simulink model "VehCtrl20260630_18B"  (R2018b)
settings: Solver=FixedStepAuto  StartTime=0.0  StopTime=inf  FixedStep=0.005  RelTol=1e-3
InitFcn:
  | mbd_mpc_consistency_checks(bdroot(gcs));
undefined symbols (not defined in the file): ANG_DEAD, BMS_NormalPwr, BrakeDeadZone, BrkPrsByBrkPct_TB_X, BrkPrsByBrkPct_TB_Y, DELAY_DISCHARGE, DELAY_RCUOFF, DRV_BACKWARD, DRV_BRAKE, DRV_FORWARD, DRV_NEUTRAL, DRV_PARK, DRV_UNPARK, DRV_ZEROTURN, EPB_LOCK, EPB_UNLOCK, ExtraLoadPwr, FanOff, fifo_0_vect, fifo_1_vect, HiFanReq, HV_finished, HV_No_Active, HV_POWER_OFF, HV_POWER_ON, HVDown, HVON, KaTLS_v_DrgUp_X_VehSpd, KeFTM_s_Way1OffDlyTime, KeFTM_TK_Way1CoolLv2OffBatTemp, KeFTM_TK_Way1CoolLv2OffMtrTemp, KeFTM_TK_Way1CoolLv2OnBatTemp, KeFTM_TK_Way1CoolLv2OnMtrTemp, KeFTM_TK_Way1CoolLv3OffBatTemp, KeFTM_TK_Way1CoolLv3OffMtrTemp, KeFTM_TK_Way1CoolLv3OnBatTemp, KeFTM_TK_Way1CoolLv3OnMtrTemp, KeFTM_TK_Way1CoolLv4OffBatTemp, KeFTM_TK_Way1CoolLv4OffMtrTemp, KeFTM_TK_Way1CoolLv4OnBatTemp, KeFTM_TK_Way1CoolLv4OnMtrTemp, Kp1, Kp2, LowFanReq, LQFP, MtrCmdGainFL, MtrCmdGainFR, MtrCmdGainRL, MtrCmdGainRR, MtrPwrFactor_RCU, MtrPwrHighToMidThd, MtrPwrLowToMidThd, MtrPwrMidToHighThd, MtrPwrMidToLowThd, MtrTrqMax, PCT_DEAD, Precharge, PTO_1000, PTO_540, pts1_fifo_0_vect ... (+32)
libraries: mbd_mpc574x_ec_toolbox x175, simulink x110, canmsglib x70
(part 6 of 15)

== system VehCtrl20260630_18B/SigIn/CAN0/RMT_VCU4 ==
  ID : Inport
  Data : Inport  Port=2
  length : Inport  Port=3
  timestamp : Inport  Port=4
  Switch Case : SwitchCase  CaseConditions={hex2dec('4')}  ShowDefaultCase=off
  UNPACK : Subsystem  TreatAsAtomicUnit=on
  Message : Outport
  wires:
  Switch Case/1 -> UNPACK/Action
  ID/1 -> UNPACK/1(ID), Switch Case/1
  Data/1 -> UNPACK/2(data)
  timestamp/1 -> UNPACK/4(timestamp)
  length/1 -> UNPACK/3(length)
  UNPACK/1(Message) -> Message/1

== system VehCtrl20260630_18B/SigIn/CAN1/ACM_Msg ==
  ID : Inport
  Data : Inport  Port=2
  length : Inport  Port=3
  timestamp : Inport  Port=4
  Switch Case : SwitchCase  CaseConditions={hex2dec('284')}  ShowDefaultCase=off
  UNPACK : Subsystem  TreatAsAtomicUnit=on
  Message : Outport
  wires:
  Switch Case/1 -> UNPACK/Action
  ID/1 -> UNPACK/1(ID), Switch Case/1
  Data/1 -> UNPACK/2(data)
  timestamp/1 -> UNPACK/4(timestamp)
  length/1 -> UNPACK/3(length)
  UNPACK/1(Message) -> Message/1

== system VehCtrl20260630_18B/SigIn/CAN1/AVCU_Msg ==
  ID : Inport
  Data : Inport  Port=2
  length : Inport  Port=3
  timestamp : Inport  Port=4
  Switch Case : SwitchCase  CaseConditions={hex2dec('180')}  ShowDefaultCase=off
  UNPACK : Subsystem  TreatAsAtomicUnit=on
  Message : Outport
  wires:
  UNPACK/1(Message) -> Message/1
  length/1 -> UNPACK/3(length)
  timestamp/1 -> UNPACK/4(timestamp)
  Data/1 -> UNPACK/2(data)
  ID/1 -> Switch Case/1, UNPACK/1(ID)
  Switch Case/1 -> UNPACK/Action

== system VehCtrl20260630_18B/SigIn/CAN1/BMS_CANWakeUpID ==
  ID : Inport
  Data : Inport  Port=2
  length : Inport  Port=3
  timestamp : Inport  Port=4
  Switch Case : SwitchCase  CaseConditions={hex2dec('180D2947')}  ShowDefaultCase=off
  UNPACK : Subsystem  TreatAsAtomicUnit=on
  Message : Outport
  wires:
  UNPACK/1(Message) -> Message/1
  length/1 -> UNPACK/3(length)
  timestamp/1 -> UNPACK/4(timestamp)
  Data/1 -> UNPACK/2(data)
  ID/1 -> Switch Case/1, UNPACK/1(ID)
  Switch Case/1 -> UNPACK/Action

== system VehCtrl20260630_18B/SigIn/CAN1/BMS_CellTempCycTx ==
  ID : Inport
  Data : Inport  Port=2
  length : Inport  Port=3
  timestamp : Inport  Port=4
  Switch Case : SwitchCase  CaseConditions={hex2dec('18602947')}  ShowDefaultCase=off
  UNPACK : Subsystem  TreatAsAtomicUnit=on
  Message : Outport
  wires:
  UNPACK/1(Message) -> Message/1
  length/1 -> UNPACK/3(length)
  timestamp/1 -> UNPACK/4(timestamp)
  Data/1 -> UNPACK/2(data)
  ID/1 -> Switch Case/1, UNPACK/1(ID)
  Switch Case/1 -> UNPACK/Action

== system VehCtrl20260630_18B/SigIn/CAN1/BMS_CellVoltageCycTx ==
  ID : Inport
  Data : Inport  Port=2
  length : Inport  Port=3
  timestamp : Inport  Port=4
  Switch Case : SwitchCase  CaseConditions={hex2dec('18202947')}  ShowDefaultCase=off
  UNPACK : Subsystem  TreatAsAtomicUnit=on
  Message : Outport
  wires:
  UNPACK/1(Message) -> Message/1
  length/1 -> UNPACK/3(length)
  timestamp/1 -> UNPACK/4(timestamp)
  Data/1 -> UNPACK/2(data)
  ID/1 -> Switch Case/1, UNPACK/1(ID)
  Switch Case/1 -> UNPACK/Action

== system VehCtrl20260630_18B/SigIn/CAN1/BMS_ExtremeCellVoltage ==
  ID : Inport
  Data : Inport  Port=2
  length : Inport  Port=3
  timestamp : Inport  Port=4
  Switch Case : SwitchCase  CaseConditions={hex2dec('18022947')}  ShowDefaultCase=off
  UNPACK : Subsystem  TreatAsAtomicUnit=on
  Message : Outport
  wires:
  UNPACK/1(Message) -> Message/1
  length/1 -> UNPACK/3(length)
  timestamp/1 -> UNPACK/4(timestamp)
  Data/1 -> UNPACK/2(data)
  ID/1 -> Switch Case/1, UNPACK/1(ID)
  Switch Case/1 -> UNPACK/Action

== system VehCtrl20260630_18B/SigIn/CAN1/BMS_ExtremeTemp ==
  ID : Inport
  Data : Inport  Port=2
  length : Inport  Port=3
  timestamp : Inport  Port=4
  Switch Case : SwitchCase  CaseConditions={hex2dec('18032947')}  ShowDefaultCase=off
  UNPACK : Subsystem  TreatAsAtomicUnit=on
  Message : Outport
  wires:
  UNPACK/1(Message) -> Message/1
  length/1 -> UNPACK/3(length)
  timestamp/1 -> UNPACK/4(timestamp)
  Data/1 -> UNPACK/2(data)
  ID/1 -> Switch Case/1, UNPACK/1(ID)
  Switch Case/1 -> UNPACK/Action

== system VehCtrl20260630_18B/SigIn/CAN1/BMS_PackCalc ==
  ID : Inport
  Data : Inport  Port=2
  length : Inport  Port=3
  timestamp : Inport  Port=4
  Switch Case : SwitchCase  CaseConditions={hex2dec('18052947')}  ShowDefaultCase=off
  UNPACK : Subsystem  TreatAsAtomicUnit=on
  Message : Outport
  wires:
  UNPACK/1(Message) -> Message/1
  length/1 -> UNPACK/3(length)
  timestamp/1 -> UNPACK/4(timestamp)
  Data/1 -> UNPACK/2(data)
  ID/1 -> Switch Case/1, UNPACK/1(ID)
  Switch Case/1 -> UNPACK/Action

== system VehCtrl20260630_18B/SigIn/CAN1/BMS_PackLimitPower ==
  ID : Inport
  Data : Inport  Port=2
  length : Inport  Port=3
  timestamp : Inport  Port=4
  Switch Case : SwitchCase  CaseConditions={hex2dec('18062947')}  ShowDefaultCase=off
  UNPACK : Subsystem  TreatAsAtomicUnit=on
  Message : Outport
  wires:
  Switch Case/1 -> UNPACK/Action
  ID/1 -> UNPACK/1(ID), Switch Case/1
  Data/1 -> UNPACK/2(data)
  timestamp/1 -> UNPACK/4(timestamp)
  length/1 -> UNPACK/3(length)
  UNPACK/1(Message) -> Message/1

== system VehCtrl20260630_18B/SigIn/CAN1/BMS_PackMeasure ==
  ID : Inport
  Data : Inport  Port=2
  length : Inport  Port=3
  timestamp : Inport  Port=4
  Switch Case : SwitchCase  CaseConditions={hex2dec('18012947')}  ShowDefaultCase=off
  UNPACK : Subsystem  TreatAsAtomicUnit=on
  Message : Outport
  wires:
  UNPACK/1(Message) -> Message/1
  length/1 -> UNPACK/3(length)
  timestamp/1 -> UNPACK/4(timestamp)
  Data/1 -> UNPACK/2(data)
  ID/1 -> Switch Case/1, UNPACK/1(ID)
  Switch Case/1 -> UNPACK/Action

== system VehCtrl20260630_18B/SigIn/CAN1/BMS_PackStateInf ==
  ID : Inport
  Data : Inport  Port=2
  length : Inport  Port=3
  timestamp : Inport  Port=4
  Switch Case : SwitchCase  CaseConditions={hex2dec('18042947')}  ShowDefaultCase=off
  UNPACK : Subsystem  TreatAsAtomicUnit=on
  Message : Outport
  wires:
  Switch Case/1 -> UNPACK/Action
  ID/1 -> UNPACK/1(ID), Switch Case/1
  Data/1 -> UNPACK/2(data)
  timestamp/1 -> UNPACK/4(timestamp)
  length/1 -> UNPACK/3(length)
  UNPACK/1(Message) -> Message/1

== system VehCtrl20260630_18B/SigIn/CAN1/BMS_Relaystatus ==
  ID : Inport
  Data : Inport  Port=2
  length : Inport  Port=3
  timestamp : Inport  Port=4
  Switch Case : SwitchCase  CaseConditions={hex2dec('1C1F7547')}  ShowDefaultCase=off
  UNPACK : Subsystem  TreatAsAtomicUnit=on
  Message : Outport
  wires:
  UNPACK/1(Message) -> Message/1
  length/1 -> UNPACK/3(length)
  timestamp/1 -> UNPACK/4(timestamp)
  Data/1 -> UNPACK/2(data)
  ID/1 -> Switch Case/1, UNPACK/1(ID)
  Switch Case/1 -> UNPACK/Action

== system VehCtrl20260630_18B/SigIn/CAN1/DbugBMS_ESM ==
  ID : Inport
  Data : Inport  Port=2
  length : Inport  Port=3
  timestamp : Inport  Port=4
  Switch Case : SwitchCase  CaseConditions={hex2dec('1C067547')}  ShowDefaultCase=off
  UNPACK : Subsystem  TreatAsAtomicUnit=on
  Message : Outport
  wires:
  UNPACK/1(Message) -> Message/1
  length/1 -> UNPACK/3(length)
  timestamp/1 -> UNPACK/4(timestamp)
  Data/1 -> UNPACK/2(data)
  ID/1 -> Switch Case/1, UNPACK/1(ID)
  Switch Case/1 -> UNPACK/Action

== system VehCtrl20260630_18B/SigIn/CAN1/DbugBMS_SOC_CaleSOC ==
  ID : Inport
  Data : Inport  Port=2
  length : Inport  Port=3
  timestamp : Inport  Port=4
  Switch Case : SwitchCase  CaseConditions={hex2dec('1C017547')}  ShowDefaultCase=off
  UNPACK : Subsystem  TreatAsAtomicUnit=on
  Message : Outport
  wires:
  Switch Case/1 -> UNPACK/Action
  ID/1 -> UNPACK/1(ID), Switch Case/1
  Data/1 -> UNPACK/2(data)
  timestamp/1 -> UNPACK/4(timestamp)
  length/1 -> UNPACK/3(length)
  UNPACK/1(Message) -> Message/1

== system VehCtrl20260630_18B/SigIn/CAN1/MCU2VCU_1 ==
  ID : Inport
  Data : Inport  Port=2
  length : Inport  Port=3
  timestamp : Inport  Port=4
  Switch Case : SwitchCase  CaseConditions={hex2dec('C08A7F3')}  ShowDefaultCase=off
  UNPACK : Subsystem  TreatAsAtomicUnit=on
  Message : Outport
  wires:
  Switch Case/1 -> UNPACK/Action
  ID/1 -> UNPACK/1(ID), Switch Case/1
  Data/1 -> UNPACK/2(data)
  timestamp/1 -> UNPACK/4(timestamp)
  length/1 -> UNPACK/3(length)
  UNPACK/1(Message) -> Message/1

== system VehCtrl20260630_18B/SigIn/CAN1/MCU2VCU_10 ==
  ID : Inport
  Data : Inport  Port=2
  length : Inport  Port=3
  timestamp : Inport  Port=4
  Switch Case : SwitchCase  CaseConditions={hex2dec('C09A7F0')}  ShowDefaultCase=off
  UNPACK : Subsystem  TreatAsAtomicUnit=on
  Message : Outport
  wires:
  Switch Case/1 -> UNPACK/Action
  ID/1 -> UNPACK/1(ID), Switch Case/1
  Data/1 -> UNPACK/2(data)
  timestamp/1 -> UNPACK/4(timestamp)
  length/1 -> UNPACK/3(length)
  UNPACK/1(Message) -> Message/1

== system VehCtrl20260630_18B/SigIn/CAN1/MCU2VCU_11 ==
  ID : Inport
  Data : Inport  Port=2
  length : Inport  Port=3
  timestamp : Inport  Port=4
  Switch Case : SwitchCase  CaseConditions={hex2dec('C0AA7F0')}  ShowDefaultCase=off
  UNPACK : Subsystem  TreatAsAtomicUnit=on
  Message : Outport
  wires:
  UNPACK/1(Message) -> Message/1
  length/1 -> UNPACK/3(length)
  timestamp/1 -> UNPACK/4(timestamp)
  Data/1 -> UNPACK/2(data)
  ID/1 -> Switch Case/1, UNPACK/1(ID)
  Switch Case/1 -> UNPACK/Action

== system VehCtrl20260630_18B/SigIn/CAN1/MCU2VCU_12 ==
  ID : Inport
  Data : Inport  Port=2
  length : Inport  Port=3
  timestamp : Inport  Port=4
  Switch Case : SwitchCase  CaseConditions={hex2dec('C0BA7F0')}  ShowDefaultCase=off
  UNPACK : Subsystem  TreatAsAtomicUnit=on
  Message : Outport
  wires:
  Switch Case/1 -> UNPACK/Action
  ID/1 -> UNPACK/1(ID), Switch Case/1
  Data/1 -> UNPACK/2(data)
  timestamp/1 -> UNPACK/4(timestamp)
  length/1 -> UNPACK/3(length)
  UNPACK/1(Message) -> Message/1

== system VehCtrl20260630_18B/SigIn/CAN1/MCU2VCU_13 ==
  ID : Inport
  Data : Inport  Port=2
  length : Inport  Port=3
  timestamp : Inport  Port=4
  Switch Case : SwitchCase  CaseConditions={hex2dec('C08A7F1')}  ShowDefaultCase=off
  UNPACK : Subsystem  TreatAsAtomicUnit=on
  Message : Outport
  wires:
  Switch Case/1 -> UNPACK/Action
  ID/1 -> UNPACK/1(ID), Switch Case/1
  Data/1 -> UNPACK/2(data)
  timestamp/1 -> UNPACK/4(timestamp)
  length/1 -> UNPACK/3(length)
  UNPACK/1(Message) -> Message/1

== system VehCtrl20260630_18B/SigIn/CAN1/MCU2VCU_14 ==
  ID : Inport
  Data : Inport  Port=2
  length : Inport  Port=3
  timestamp : Inport  Port=4
  Switch Case : SwitchCase  CaseConditions={hex2dec('C09A7F1')}  ShowDefaultCase=off
  UNPACK : Subsystem  TreatAsAtomicUnit=on
  Message : Outport
  wires:
  UNPACK/1(Message) -> Message/1
  length/1 -> UNPACK/3(length)
  timestamp/1 -> UNPACK/4(timestamp)
  Data/1 -> UNPACK/2(data)
  ID/1 -> Switch Case/1, UNPACK/1(ID)
  Switch Case/1 -> UNPACK/Action

== system VehCtrl20260630_18B/SigIn/CAN1/MCU2VCU_15 ==
  ID : Inport
  Data : Inport  Port=2
  length : Inport  Port=3
  timestamp : Inport  Port=4
  Switch Case : SwitchCase  CaseConditions={hex2dec('C0AA7F1')}  ShowDefaultCase=off
  UNPACK : Subsystem  TreatAsAtomicUnit=on
  Message : Outport
  wires:
  Switch Case/1 -> UNPACK/Action
  ID/1 -> UNPACK/1(ID), Switch Case/1
  Data/1 -> UNPACK/2(data)
  timestamp/1 -> UNPACK/4(timestamp)
  length/1 -> UNPACK/3(length)
  UNPACK/1(Message) -> Message/1

== system VehCtrl20260630_18B/SigIn/CAN1/MCU2VCU_16 ==
  ID : Inport
  Data : Inport  Port=2
  length : Inport  Port=3
  timestamp : Inport  Port=4
  Switch Case : SwitchCase  CaseConditions={hex2dec('C0BA7F1')}  ShowDefaultCase=off
  UNPACK : Subsystem  TreatAsAtomicUnit=on
  Message : Outport
  wires:
  UNPACK/1(Message) -> Message/1
  length/1 -> UNPACK/3(length)
  timestamp/1 -> UNPACK/4(timestamp)
  Data/1 -> UNPACK/2(data)
  ID/1 -> Switch Case/1, UNPACK/1(ID)
  Switch Case/1 -> UNPACK/Action

== system VehCtrl20260630_18B/SigIn/CAN1/MCU2VCU_17 ==
  ID : Inport
  Data : Inport  Port=2
  length : Inport  Port=3
  timestamp : Inport  Port=4
  Switch Case : SwitchCase  CaseConditions={hex2dec('C08A7F4')}  ShowDefaultCase=off
  UNPACK : Subsystem  TreatAsAtomicUnit=on
  Message : Outport
  wires:
  Switch Case/1 -> UNPACK/Action
  ID/1 -> UNPACK/1(ID), Switch Case/1
  Data/1 -> UNPACK/2(data)
  timestamp/1 -> UNPACK/4(timestamp)
  length/1 -> UNPACK/3(length)
  UNPACK/1(Message) -> Message/1

== system VehCtrl20260630_18B/SigIn/CAN1/MCU2VCU_18 ==
  ID : Inport
  Data : Inport  Port=2
  length : Inport  Port=3
  timestamp : Inport  Port=4
  Switch Case : SwitchCase  CaseConditions={hex2dec('C09A7F4')}  ShowDefaultCase=off
  UNPACK : Subsystem  TreatAsAtomicUnit=on
  Message : Outport
  wires:
  Switch Case/1 -> UNPACK/Action
  ID/1 -> UNPACK/1(ID), Switch Case/1
  Data/1 -> UNPACK/2(data)
  timestamp/1 -> UNPACK/4(timestamp)
  length/1 -> UNPACK/3(length)
  UNPACK/1(Message) -> Message/1

== system VehCtrl20260630_18B/SigIn/CAN1/MCU2VCU_19 ==
  ID : Inport
  Data : Inport  Port=2
  length : Inport  Port=3
  timestamp : Inport  Port=4
  Switch Case : SwitchCase  CaseConditions={hex2dec('C0AA7F4')}  ShowDefaultCase=off
  UNPACK : Subsystem  TreatAsAtomicUnit=on
  Message : Outport
  wires:
  UNPACK/1(Message) -> Message/1
  length/1 -> UNPACK/3(length)
  timestamp/1 -> UNPACK/4(timestamp)
  Data/1 -> UNPACK/2(data)
  ID/1 -> Switch Case/1, UNPACK/1(ID)
  Switch Case/1 -> UNPACK/Action

== system VehCtrl20260630_18B/SigIn/CAN1/MCU2VCU_2 ==
  ID : Inport
  Data : Inport  Port=2
  length : Inport  Port=3
  timestamp : Inport  Port=4
  Switch Case : SwitchCase  CaseConditions={hex2dec('C09A7F3')}  ShowDefaultCase=off
  UNPACK : Subsystem  TreatAsAtomicUnit=on
  Message : Outport
  wires:
  UNPACK/1(Message) -> Message/1
  length/1 -> UNPACK/3(length)
  timestamp/1 -> UNPACK/4(timestamp)
  Data/1 -> UNPACK/2(data)
  ID/1 -> Switch Case/1, UNPACK/1(ID)
  Switch Case/1 -> UNPACK/Action

== system VehCtrl20260630_18B/SigIn/CAN1/MCU2VCU_20 ==
  ID : Inport
  Data : Inport  Port=2
  length : Inport  Port=3
  timestamp : Inport  Port=4
  Switch Case : SwitchCase  CaseConditions={hex2dec('C0BA7F4')}  ShowDefaultCase=off
  UNPACK : Subsystem  TreatAsAtomicUnit=on
  Message : Outport
  wires:
  Switch Case/1 -> UNPACK/Action
  ID/1 -> UNPACK/1(ID), Switch Case/1
  Data/1 -> UNPACK/2(data)
  timestamp/1 -> UNPACK/4(timestamp)
  length/1 -> UNPACK/3(length)
  UNPACK/1(Message) -> Message/1

== system VehCtrl20260630_18B/SigIn/CAN1/MCU2VCU_3 ==
  ID : Inport
  Data : Inport  Port=2
  length : Inport  Port=3
  timestamp : Inport  Port=4
  Switch Case : SwitchCase  CaseConditions={hex2dec('C0AA7F3')}  ShowDefaultCase=off
  UNPACK : Subsystem  TreatAsAtomicUnit=on
  Message : Outport
  wires:
  Switch Case/1 -> UNPACK/Action
  ID/1 -> UNPACK/1(ID), Switch Case/1
  Data/1 -> UNPACK/2(data)
  timestamp/1 -> UNPACK/4(timestamp)
  length/1 -> UNPACK/3(length)
  UNPACK/1(Message) -> Message/1

== system VehCtrl20260630_18B/SigIn/CAN1/MCU2VCU_4 ==
  ID : Inport
  Data : Inport  Port=2
  length : Inport  Port=3
  timestamp : Inport  Port=4
  Switch Case : SwitchCase  CaseConditions={hex2dec('C0BA7F3')}  ShowDefaultCase=off
  UNPACK : Subsystem  TreatAsAtomicUnit=on
  Message : Outport
  wires:
  UNPACK/1(Message) -> Message/1
  length/1 -> UNPACK/3(length)
  timestamp/1 -> UNPACK/4(timestamp)
  Data/1 -> UNPACK/2(data)
  ID/1 -> Switch Case/1, UNPACK/1(ID)
  Switch Case/1 -> UNPACK/Action

== system VehCtrl20260630_18B/SigIn/CAN1/MCU2VCU_5 ==
  ID : Inport
  Data : Inport  Port=2
  length : Inport  Port=3
  timestamp : Inport  Port=4
  Switch Case : SwitchCase  CaseConditions={hex2dec('C08A7F2')}  ShowDefaultCase=off
  UNPACK : Subsystem  TreatAsAtomicUnit=on
  Message : Outport
  wires:
  Switch Case/1 -> UNPACK/Action
  ID/1 -> UNPACK/1(ID), Switch Case/1
  Data/1 -> UNPACK/2(data)
  timestamp/1 -> UNPACK/4(timestamp)
  length/1 -> UNPACK/3(length)
  UNPACK/1(Message) -> Message/1

== system VehCtrl20260630_18B/SigIn/CAN1/MCU2VCU_6 ==
  ID : Inport
  Data : Inport  Port=2
  length : Inport  Port=3
  timestamp : Inport  Port=4
  Switch Case : SwitchCase  CaseConditions={hex2dec('C09A7F2')}  ShowDefaultCase=off
  UNPACK : Subsystem  TreatAsAtomicUnit=on
  Message : Outport
  wires:
  Switch Case/1 -> UNPACK/Action
  ID/1 -> UNPACK/1(ID), Switch Case/1
  Data/1 -> UNPACK/2(data)
  timestamp/1 -> UNPACK/4(timestamp)
  length/1 -> UNPACK/3(length)
  UNPACK/1(Message) -> Message/1

== system VehCtrl20260630_18B/SigIn/CAN1/MCU2VCU_7 ==
  ID : Inport
  Data : Inport  Port=2
  length : Inport  Port=3
  timestamp : Inport  Port=4
  Switch Case : SwitchCase  CaseConditions={hex2dec('C0AA7F2')}  ShowDefaultCase=off
  UNPACK : Subsystem  TreatAsAtomicUnit=on
  Message : Outport
  wires:
  UNPACK/1(Message) -> Message/1
  length/1 -> UNPACK/3(length)
  timestamp/1 -> UNPACK/4(timestamp)
  Data/1 -> UNPACK/2(data)
  ID/1 -> Switch Case/1, UNPACK/1(ID)
  Switch Case/1 -> UNPACK/Action

== system VehCtrl20260630_18B/SigIn/CAN1/MCU2VCU_8 ==
  ID : Inport
  Data : Inport  Port=2
  length : Inport  Port=3
  timestamp : Inport  Port=4
  Switch Case : SwitchCase  CaseConditions={hex2dec('C0BA7F2')}  ShowDefaultCase=off
  UNPACK : Subsystem  TreatAsAtomicUnit=on
  Message : Outport
  wires:
  Switch Case/1 -> UNPACK/Action
  ID/1 -> UNPACK/1(ID), Switch Case/1
  Data/1 -> UNPACK/2(data)
  timestamp/1 -> UNPACK/4(timestamp)
  length/1 -> UNPACK/3(length)
  UNPACK/1(Message) -> Message/1

== system VehCtrl20260630_18B/SigIn/CAN1/MCU2VCU_9 ==
  ID : Inport
  Data : Inport  Port=2
  length : Inport  Port=3
  timestamp : Inport  Port=4
  Switch Case : SwitchCase  CaseConditions={hex2dec('C08A7F0')}  ShowDefaultCase=off
  UNPACK : Subsystem  TreatAsAtomicUnit=on
  Message : Outport
  wires:
  Switch Case/1 -> UNPACK/Action
  ID/1 -> UNPACK/1(ID), Switch Case/1
  Data/1 -> UNPACK/2(data)
  timestamp/1 -> UNPACK/4(timestamp)
  length/1 -> UNPACK/3(length)
  UNPACK/1(Message) -> Message/1

== system VehCtrl20260630_18B/SigIn/CAN1/RCU_MSG_1 ==
  ID : Inport
  Data : Inport  Port=2
  length : Inport  Port=3
  timestamp : Inport  Port=4
  Switch Case : SwitchCase  CaseConditions={hex2dec('18F0011B')}  ShowDefaultCase=off
  UNPACK : Subsystem  TreatAsAtomicUnit=on
  Message : Outport
  wires:
  Switch Case/1 -> UNPACK/Action
  ID/1 -> UNPACK/1(ID), Switch Case/1
  Data/1 -> UNPACK/2(data)
  timestamp/1 -> UNPACK/4(timestamp)
  length/1 -> UNPACK/3(length)
  UNPACK/1(Message) -> Message/1

== system VehCtrl20260630_18B/SigIn/CAN1/RCU_MSG_2 ==
  ID : Inport
  Data : Inport  Port=2
  length : Inport  Port=3
  timestamp : Inport  Port=4
  Switch Case : SwitchCase  CaseConditions={hex2dec('18F0022B')}  ShowDefaultCase=off
  UNPACK : Subsystem  TreatAsAtomicUnit=on
  Message : Outport
  wires:
  UNPACK/1(Message) -> Message/1
  length/1 -> UNPACK/3(length)
  timestamp/1 -> UNPACK/4(timestamp)
  Data/1 -> UNPACK/2(data)
  ID/1 -> Switch Case/1, UNPACK/1(ID)
  Switch Case/1 -> UNPACK/Action

== system VehCtrl20260630_18B/SigIn/CAN1/RCU_MSG_3 ==
  ID : Inport
  Data : Inport  Port=2
  length : Inport  Port=3
  timestamp : Inport  Port=4
  Switch Case : SwitchCase  CaseConditions={hex2dec('18F0033B')}  ShowDefaultCase=off
  UNPACK : Subsystem  TreatAsAtomicUnit=on
  Message : Outport
  wires:
  Switch Case/1 -> UNPACK/Action
  ID/1 -> UNPACK/1(ID), Switch Case/1
  Data/1 -> UNPACK/2(data)
  timestamp/1 -> UNPACK/4(timestamp)
  length/1 -> UNPACK/3(length)
  UNPACK/1(Message) -> Message/1

== system VehCtrl20260630_18B/SigIn/CAN1/SENSOR_Msg ==
  ID : Inport
  Data : Inport  Port=2
  length : Inport  Port=3
  timestamp : Inport  Port=4
  Switch Case : SwitchCase  CaseConditions={hex2dec('585')}  ShowDefaultCase=off
  UNPACK : Subsystem  TreatAsAtomicUnit=on
  Message : Outport
  wires:
  Switch Case/1 -> UNPACK/Action
  ID/1 -> UNPACK/1(ID), Switch Case/1
  Data/1 -> UNPACK/2(data)
  timestamp/1 -> UNPACK/4(timestamp)
  length/1 -> UNPACK/3(length)
  UNPACK/1(Message) -> Message/1

== system VehCtrl20260630_18B/SigIn/DI/DI_31_32_33_34 ==
  note: DI PWM PULLUP
  note: DI PWM PULLDOWN
  DI31 : mbd_mpc574x_ec_toolbox/GPIO Blocks/Digital_Input  gpio_pin=PTF0: [SIUL2_GPIO80 | General Purpose IO PF[0]]  pull_resistor=None
  DI32 : mbd_mpc574x_ec_toolbox/GPIO Blocks/Digital_Input  gpio_pin=PTD1: [SIUL2_GPIO49 | General Purpose IO PD[1]]  pull_resistor=None
  DI33 : mbd_mpc574x_ec_toolbox/GPIO Blocks/Digital_Input  gpio_pin=PTD2: [SIUL2_GPIO50 | General Purpose IO PD[2]]  pull_resistor=None
  DI34 : mbd_mpc574x_ec_toolbox/GPIO Blocks/Digital_Input  gpio_pin=PTC13: [SIUL2_GPIO45 | General Purpose IO PC[13]]  pull_resistor=None
  Data Store Write14 : DataStoreWrite  DataStoreName=DI31
  Data Store Write15 : DataStoreWrite  DataStoreName=DI32
  Data Store Write16 : DataStoreWrite  DataStoreName=DI33
  Data Store Write17 : DataStoreWrite  DataStoreName=DI34
  wires:
  DI34/1 -> Data Store Write17/1
  DI33/1 -> Data Store Write16/1
  DI32/1 -> Data Store Write15/1
  DI31/1 -> Data Store Write14/1

== system VehCtrl20260630_18B/SigIn/PWM/PWM_PTS1 ==
  Add : Sum  Inputs=+-  AccumDataTypeStr=single
  Add1 : Sum  Inputs=+-  AccumDataTypeStr=single
  Data Store Memory : DataStoreMemory  DataStoreName=pts1_pwm_cnt  ReadBeforeWriteMsg=warning  WriteAfterWriteMsg=warning  WriteAfterReadMsg=warning  ShowAdditionalParam=off  OutDataTypeStr=uint8
  Data Store Memory2 : DataStoreMemory  DataStoreName=pts1_fifo_1_vect  ReadBeforeWriteMsg=warning  WriteAfterWriteMsg=warning  WriteAfterReadMsg=warning  InitialValue=[0 0 0 0 0 0 0 0]  ShowAdditionalParam=off  OutDataTypeStr=uint16
  Data Store Memory4 : DataStoreMemory  DataStoreName=pts1_fifo_0_vect  ReadBeforeWriteMsg=warning  WriteAfterWriteMsg=warning  WriteAfterReadMsg=warning  InitialValue=[0 0 0 0 0 0 0 0]  ShowAdditionalParam=off  OutDataTypeStr=uint16
  Data Store Read : DataStoreRead  DataStoreName=pts1_fifo_0_vect  DataStoreElements=pts1_fifo_0_vect(2)#pts1_fifo_0_vect(1)
  Data Store Read1 : DataStoreRead  DataStoreName=pts1_fifo_1_vect  DataStoreElements=pts1_fifo_1_vect(1)
  Data Store Read2 : DataStoreRead  DataStoreName=pts1_fifo_0_vect  DataStoreElements=pts1_fifo_0_vect(1)
  Data Store Write3 : DataStoreWrite  DataStoreName=pts1_fifo_0_vect
  Data Store Write5 : DataStoreWrite  DataStoreName=pts1_fifo_1_vect
  Divide : Product  Inputs=*/  OutDataTypeStr=single
  Divide1 : Product  Inputs=*//
  Freq_MC : Constant  Value=80000000  OutDataTypeStr=single
  Prescaler : Constant  Value=32  OutDataTypeStr=single
  Subsystem : Subsystem
  Subsystem_capture : Subsystem
  Terminator1 : Terminator
  Terminator2 : Terminator
  eTimer_ISR : mbd_mpc574x_ec_toolbox/Motor Control Blocks/eTIMER Blocks/eTimer_ISR_Handler  etimerModule=1  etimerInterrupt=Channel Interrupt  etimerChannel=2  etimerIsrPriority=14
      settings: SourceProductName=NXP Model-Based Design Toolbox for MPC57xx MCUs
  DC : Outport
  freq : Outport  Port=2
  wires:
  eTimer_ISR/2 -> Subsystem_capture/1(In1)
  Subsystem_capture/1(Out1) -> Terminator1/1
  Subsystem_capture/3(Out3) -> Terminator2/1
  Subsystem_capture/4(Out4) -> Data Store Write5/1
  Subsystem_capture/2(Out2) -> Data Store Write3/1
  eTimer_ISR/1 -> Subsystem_capture/Trigger
  Prescaler/1 -> Divide1/2
  Add/1 -> Divide/2, Divide1/3
  Data Store Read1/1 -> Add1/1
  Data Store Read/2 -> Add/2
  Freq_MC/1 -> Divide1/1
  Add1/1 -> Divide/1
  Data Store Read2/1 -> Add1/2
  Divide1/1 -> freq/1
  Data Store Read/1 -> Add/1
  Divide/1 -> Subsystem/1(In1)
  Subsystem/1(Out1) -> DC/1

== system VehCtrl20260630_18B/SigIn/PWM/PWM_PTS2 ==
  Add : Sum  Inputs=+-  AccumDataTypeStr=single
  Add1 : Sum  Inputs=+-  AccumDataTypeStr=single
  Data Store Memory : DataStoreMemory  DataStoreName=pts2_pwm_cnt  ReadBeforeWriteMsg=warning  WriteAfterWriteMsg=warning  WriteAfterReadMsg=warning  ShowAdditionalParam=off  OutDataTypeStr=uint8
  Data Store Memory2 : DataStoreMemory  DataStoreName=pts2_fifo_1_vect  ReadBeforeWriteMsg=warning  WriteAfterWriteMsg=warning  WriteAfterReadMsg=warning  InitialValue=[0 0 0 0 0 0 0 0]  ShowAdditionalParam=off  OutDataTypeStr=uint16
  Data Store Memory4 : DataStoreMemory  DataStoreName=pts2_fifo_0_vect  ReadBeforeWriteMsg=warning  WriteAfterWriteMsg=warning  WriteAfterReadMsg=warning  InitialValue=[0 0 0 0 0 0 0 0]  ShowAdditionalParam=off  OutDataTypeStr=uint16
  Data Store Read : DataStoreRead  DataStoreName=pts2_fifo_0_vect  DataStoreElements=pts2_fifo_0_vect(2)#pts2_fifo_0_vect(1)
  Data Store Read1 : DataStoreRead  DataStoreName=pts2_fifo_1_vect  DataStoreElements=pts2_fifo_1_vect(1)
  Data Store Read2 : DataStoreRead  DataStoreName=pts2_fifo_0_vect  DataStoreElements=pts2_fifo_0_vect(1)
  Data Store Write3 : DataStoreWrite  DataStoreName=pts2_fifo_0_vect
  Data Store Write5 : DataStoreWrite  DataStoreName=pts2_fifo_1_vect
  Divide : Product  Inputs=*/  OutDataTypeStr=single
  Divide1 : Product  Inputs=*//
  Freq_MC : Constant  Value=80000000  OutDataTypeStr=single
  Prescaler : Constant  Value=32  OutDataTypeStr=single
  Subsystem : Subsystem
  Subsystem_capture : Subsystem
  Terminator1 : Terminator
  Terminator2 : Terminator
  eTimer_ISR : mbd_mpc574x_ec_toolbox/Motor Control Blocks/eTIMER Blocks/eTimer_ISR_Handler  etimerModule=1  etimerInterrupt=Channel Interrupt  etimerChannel=3  etimerIsrPriority=14
      settings: SourceProductName=NXP Model-Based Design Toolbox for MPC57xx MCUs
  DC : Outport
  freq : Outport  Port=2
  wires:
  Subsystem/1(Out1) -> DC/1
  Divide/1 -> Subsystem/1(In1)
  Data Store Read/1 -> Add/1
  Divide1/1 -> freq/1
  Data Store Read2/1 -> Add1/2
  Add1/1 -> Divide/1
  Freq_MC/1 -> Divide1/1
  Data Store Read/2 -> Add/2
  Data Store Read1/1 -> Add1/1
  Add/1 -> Divide1/3, Divide/2
  Prescaler/1 -> Divide1/2
  eTimer_ISR/1 -> Subsystem_capture/Trigger
  Subsystem_capture/2(Out2) -> Data Store Write3/1
  Subsystem_capture/4(Out4) -> Data Store Write5/1
  Subsystem_capture/3(Out3) -> Terminator2/1
  Subsystem_capture/1(Out1) -> Terminator1/1
  eTimer_ISR/2 -> Subsystem_capture/1(In1)

== system VehCtrl20260630_18B/SigIn/PWM/PWM_PTS3 ==
  Add : Sum  Inputs=+-  AccumDataTypeStr=single
  Add1 : Sum  Inputs=+-  AccumDataTypeStr=single
  Data Store Memory : DataStoreMemory  DataStoreName=pts3_pwm_cnt  ReadBeforeWriteMsg=warning  WriteAfterWriteMsg=warning  WriteAfterReadMsg=warning  ShowAdditionalParam=off  OutDataTypeStr=uint8
  Data Store Memory2 : DataStoreMemory  DataStoreName=pts3_fifo_1_vect  ReadBeforeWriteMsg=warning  WriteAfterWriteMsg=warning  WriteAfterReadMsg=warning  InitialValue=[0 0 0 0 0 0 0 0]  ShowAdditionalParam=off  OutDataTypeStr=uint16
  Data Store Memory4 : DataStoreMemory  DataStoreName=pts3_fifo_0_vect  ReadBeforeWriteMsg=warning  WriteAfterWriteMsg=warning  WriteAfterReadMsg=warning  InitialValue=[0 0 0 0 0 0 0 0]  ShowAdditionalParam=off  OutDataTypeStr=uint16
  Data Store Read : DataStoreRead  DataStoreName=pts3_fifo_0_vect  DataStoreElements=pts3_fifo_0_vect(2)#pts3_fifo_0_vect(1)
  Data Store Read1 : DataStoreRead  DataStoreName=pts3_fifo_1_vect  DataStoreElements=pts3_fifo_1_vect(1)
  Data Store Read2 : DataStoreRead  DataStoreName=pts3_fifo_0_vect  DataStoreElements=pts3_fifo_0_vect(1)
  Data Store Write3 : DataStoreWrite  DataStoreName=pts3_fifo_0_vect
  Data Store Write5 : DataStoreWrite  DataStoreName=pts3_fifo_1_vect
  Divide : Product  Inputs=*/  OutDataTypeStr=single
  Divide1 : Product  Inputs=*//
  Freq_MC : Constant  Value=80000000  OutDataTypeStr=single
  Prescaler : Constant  Value=32  OutDataTypeStr=single
  Subsystem : Subsystem
  Subsystem_capture : Subsystem
  Terminator1 : Terminator
  Terminator2 : Terminator
  eTimer_ISR : mbd_mpc574x_ec_toolbox/Motor Control Blocks/eTIMER Blocks/eTimer_ISR_Handler  etimerModule=1  etimerInterrupt=Channel Interrupt  etimerChannel=1  etimerIsrPriority=14
      settings: SourceProductName=NXP Model-Based Design Toolbox for MPC57xx MCUs
  DC : Outport
  freq : Outport  Port=2
  wires:
  eTimer_ISR/2 -> Subsystem_capture/1(In1)
  Subsystem_capture/1(Out1) -> Terminator1/1
  Subsystem_capture/3(Out3) -> Terminator2/1
  Subsystem_capture/4(Out4) -> Data Store Write5/1
  Subsystem_capture/2(Out2) -> Data Store Write3/1
  eTimer_ISR/1 -> Subsystem_capture/Trigger
  Prescaler/1 -> Divide1/2
  Add/1 -> Divide/2, Divide1/3
  Data Store Read1/1 -> Add1/1
  Data Store Read/2 -> Add/2
  Freq_MC/1 -> Divide1/1
  Add1/1 -> Divide/1
  Data Store Read2/1 -> Add1/2
  Divide1/1 -> freq/1
  Data Store Read/1 -> Add/1
  Divide/1 -> Subsystem/1(In1)
  Subsystem/1(Out1) -> DC/1

== system VehCtrl20260630_18B/SigIn/PWM/PWM_PTS4 ==
  Add : Sum  Inputs=+-  AccumDataTypeStr=single
  Add1 : Sum  Inputs=+-  AccumDataTypeStr=single
  Data Store Memory : DataStoreMemory  DataStoreName=pts4_pwm_cnt  ReadBeforeWriteMsg=warning  WriteAfterWriteMsg=warning  WriteAfterReadMsg=warning  ShowAdditionalParam=off  OutDataTypeStr=uint8
  Data Store Memory2 : DataStoreMemory  DataStoreName=pts4_fifo_1_vect  ReadBeforeWriteMsg=warning  WriteAfterWriteMsg=warning  WriteAfterReadMsg=warning  InitialValue=[0 0 0 0 0 0 0 0]  ShowAdditionalParam=off  OutDataTypeStr=uint16
  Data Store Memory4 : DataStoreMemory  DataStoreName=pts4_fifo_0_vect  ReadBeforeWriteMsg=warning  WriteAfterWriteMsg=warning  WriteAfterReadMsg=warning  InitialValue=[0 0 0 0 0 0 0 0]  ShowAdditionalParam=off  OutDataTypeStr=uint16
  Data Store Read : DataStoreRead  DataStoreName=pts4_fifo_0_vect  DataStoreElements=pts4_fifo_0_vect(2)#pts4_fifo_0_vect(1)
  Data Store Read1 : DataStoreRead  DataStoreName=pts4_fifo_1_vect  DataStoreElements=pts4_fifo_1_vect(1)
  Data Store Read2 : DataStoreRead  DataStoreName=pts4_fifo_0_vect  DataStoreElements=pts4_fifo_0_vect(1)
  Data Store Write3 : DataStoreWrite  DataStoreName=pts4_fifo_0_vect
  Data Store Write5 : DataStoreWrite  DataStoreName=pts4_fifo_1_vect
  Divide : Product  Inputs=*/  OutDataTypeStr=single
  Divide1 : Product  Inputs=*//
  Freq_MC : Constant  Value=80000000  OutDataTypeStr=single
  Prescaler : Constant  Value=32  OutDataTypeStr=single
  Subsystem : Subsystem
  Subsystem_capture : Subsystem
  Terminator1 : Terminator
  Terminator2 : Terminator
  eTimer_ISR : mbd_mpc574x_ec_toolbox/Motor Control Blocks/eTIMER Blocks/eTimer_ISR_Handler  etimerModule=0  etimerInterrupt=Channel Interrupt  etimerChannel=2  etimerIsrPriority=14
      settings: SourceProductName=NXP Model-Based Design Toolbox for MPC57xx MCUs
  DC : Outport
  freq : Outport  Port=2
  wires:
  Subsystem/1(Out1) -> DC/1
  Divide/1 -> Subsystem/1(In1)
  Data Store Read/1 -> Add/1
  Divide1/1 -> freq/1
  Data Store Read2/1 -> Add1/2
  Add1/1 -> Divide/1
  Freq_MC/1 -> Divide1/1
  Data Store Read/2 -> Add/2
  Data Store Read1/1 -> Add1/1
  Add/1 -> Divide1/3, Divide/2
  Prescaler/1 -> Divide1/2
  eTimer_ISR/1 -> Subsystem_capture/Trigger
  Subsystem_capture/2(Out2) -> Data Store Write3/1
  Subsystem_capture/4(Out4) -> Data Store Write5/1
  Subsystem_capture/3(Out3) -> Terminator2/1
  Subsystem_capture/1(Out1) -> Terminator1/1
  eTimer_ISR/2 -> Subsystem_capture/1(In1)

== system VehCtrl20260630_18B/SigIn/PWM/Subsystem ==
  Data Store Memory1 : DataStoreMemory  DataStoreName=fifo_1_value  ReadBeforeWriteMsg=warning  WriteAfterWriteMsg=warning  WriteAfterReadMsg=warning  VectorParams1D=off  ShowAdditionalParam=off  OutDataTypeStr=uint16
  Data Store Memory3 : DataStoreMemory  DataStoreName=fifo_0_value  ReadBeforeWriteMsg=warning  WriteAfterWriteMsg=warning  WriteAfterReadMsg=warning  VectorParams1D=off  ShowAdditionalParam=off  OutDataTypeStr=uint16
  Data Store Memory5 : DataStoreMemory  DataStoreName=frequency  ReadBeforeWriteMsg=warning  WriteAfterWriteMsg=warning  WriteAfterReadMsg=warning  VectorParams1D=off  ShowAdditionalParam=off  OutDataTypeStr=single
  Data Store Memory6 : DataStoreMemory  DataStoreName=duty_cycle  ReadBeforeWriteMsg=warning  WriteAfterWriteMsg=warning  WriteAfterReadMsg=warning  VectorParams1D=off  ShowAdditionalParam=off  OutDataTypeStr=single
  Data Store Write10 : DataStoreWrite  DataStoreName=fifo_0_vect
  Data Store Write11 : DataStoreWrite  DataStoreName=fifo_1_value
  Data Store Write12 : DataStoreWrite  DataStoreName=fifo_1_vect
  Data Store Write13 : DataStoreWrite  DataStoreName=duty_cycle
  Data Store Write8 : DataStoreWrite  DataStoreName=frequency
  Data Store Write9 : DataStoreWrite  DataStoreName=fifo_0_value
  Frequency_DutyCycle_Computation : Subsystem
  eTimer Configuration and Signal Measurements : Subsystem
  wires:
  eTimer Configuration and Signal Measurements/4(Out4) -> Data Store Write12/1
  eTimer Configuration and Signal Measurements/2(Out2) -> Data Store Write10/1
  eTimer Configuration and Signal Measurements/3(Out3) -> Data Store Write11/1
  eTimer Configuration and Signal Measurements/1(Out1) -> Data Store Write9/1
  Frequency_DutyCycle_Computation/2(Out2) -> Data Store Write8/1
  Frequency_DutyCycle_Computation/1(Out1) -> Data Store Write13/1

== system VehCtrl20260630_18B/SigOut/AUTO/Subsystem ==
  "Press " : Inport
  fault : Inport  Port=2
  Compare To Constant1 : simulink/Logic and Bit Operations/Compare To Constant  relop=>  const=BrakeDeadZone  OutDataTypeStr=boolean
  Constant : Constant  Value=2  OutDataTypeStr=uint8
  Data Type Conversion : DataTypeConversion  OutDataTypeStr=uint8
  Switch : Switch  Criteria=u2 ~= 0
  Out1 : Outport
  wires:
  "Press "/1 -> Compare To Constant1/1
  Compare To Constant1/1 -> Data Type Conversion/1
  fault/1 -> Switch/2
  Constant/1 -> Switch/1
  Data Type Conversion/1 -> Switch/3
  Switch/1 -> Out1/1

== system VehCtrl20260630_18B/SigOut/AUTO/Subsystem1 ==
  Constant : Constant  Value=2
  Data Store Read1 : DataStoreRead  DataStoreName=CtrMode
  Data Store Read2 : DataStoreRead  DataStoreName=Fault
  Data Type Conversion : DataTypeConversion
  Data Type Conversion1 : DataTypeConversion
  Switch : Switch  Criteria=u2 > Threshold
  Out1 : Outport
  wires:
  Switch/1 -> Data Type Conversion1/1
  Data Store Read2/1 -> Switch/2
  Data Store Read1/1 -> Data Type Conversion/1
  Constant/1 -> Switch/1
  Data Type Conversion/1 -> Switch/3
  Data Type Conversion1/1 -> Out1/1

== system VehCtrl20260630_18B/SigOut/GPIO /ETC ==
  note: CMPLD1 - low
      | CMPLD2 - high
      | CMPLD1 + CMPLD2 = frequency
      | example:
      | 10kHz @50%: CMPLD1=4000, CMPLD2=4000
      | 10kHz @25%: CMPLD1=2000, CMPLD2=6000
      | 20kHz @25%: CMPLD1=1000, CMPLD2=3000
      |
      | 不控频率，固定10kHz
  note: LS ETC
  note: LS ETC
  Add1 : Sum  Inputs=-+
  Add2 : Sum  Inputs=-+
  Add3 : Sum  Inputs=-+
  Add4 : Sum  Commented=on  Inputs=-+
  Add5 : Sum  Commented=on  Inputs=-+
  Add6 : Sum  Commented=on  Inputs=-+
  Data Store Read : DataStoreRead  Commented=on  DataStoreName=HS008_ETC_DC
  Data Store Read1 : DataStoreRead  DataStoreName=LSO17_ETC_DC
  Data Store Read12 : DataStoreRead  DataStoreName=LSO18_ETC_DC
  Data Store Read13 : DataStoreRead  DataStoreName=LSO18_ETC_FRQ
  Data Store Read2 : DataStoreRead  Commented=on  DataStoreName=HS014_ETC_DC
  Data Store Read3 : DataStoreRead  DataStoreName=LSO17_ETC_FRQ
  Data Store Read4 : DataStoreRead  DataStoreName=LSO3_ETC_DC
  Data Store Read5 : DataStoreRead  DataStoreName=LSO3_ETC_FRQ
  Data Store Read6 : DataStoreRead  Commented=on  DataStoreName=LSO19_ETC_DC
  Data Store Read7 : DataStoreRead  Commented=on  DataStoreName=HSO14_ETC_FRQ
  Data Store Read8 : DataStoreRead  Commented=on  DataStoreName=LSO19_ETC_FRQ
  Data Store Read9 : DataStoreRead  Commented=on  DataStoreName=HS008_ETC_FRQ
  Divide : Product  Commented=on  Inputs=*//
  Divide1 : Product  Commented=on  Inputs=*//
  Divide2 : Product  Inputs=*//
  Divide3 : Product  Inputs=*//
  Divide4 : Product  Inputs=*//
  Divide6 : Product  Commented=on  Inputs=*//
  Freq_MC : Constant  Commented=on  Value=80000000  OutDataTypeStr=single
  Freq_MC1 : Constant  Commented=on  Value=80000000  OutDataTypeStr=single
  Freq_MC2 : Constant  Commented=on  Value=80000000  OutDataTypeStr=single
  Freq_MC3 : Constant  Value=80000000  OutDataTypeStr=single
  Freq_MC4 : Constant  Value=80000000  OutDataTypeStr=single
  Freq_MC5 : Constant  Value=80000000  OutDataTypeStr=single
  Pre : Constant  Commented=on  Value=64
  Pre1 : Constant  Commented=on  Value=64
  Pre2 : Constant  Commented=on  Value=64
  Pre3 : Constant  Value=64
  Pre4 : Constant  Value=64
  Pre5 : Constant  Value=64
  Product1 : Product
  Product2 : Product
  Product3 : Product  Commented=on
  Product4 : Product  Commented=on
  Product5 : Product  Commented=on
  Product6 : Product
  Subsystem : Subsystem
  Subsystem1 : Subsystem
  Subsystem2 : Subsystem
  Subsystem3 : Subsystem  Commented=on
  Subsystem4 : Subsystem  Commented=on
  Subsystem5 : Subsystem  Commented=on
  wires:
  Data Store Read6/1 -> Product5/1
  Product5/1 -> Add5/1, Subsystem5/1(COMPLD1)
  Add5/1 -> Subsystem5/2(COMPLD2)
  Add4/1 -> Subsystem4/2(COMPLD2)
  Data Store Read8/1 -> Divide/3
  Data Store Read2/1 -> Product4/1
  Freq_MC/1 -> Divide/1
  Divide/1 -> Product5/2, Add5/2
  Divide6/1 -> Product4/2, Add4/2
  Freq_MC1/1 -> Divide6/1
  Data Store Read7/1 -> Divide6/3
  Product4/1 -> Add4/1, Subsystem4/1(COMPLD1)
  Divide1/1 -> Product3/2, Add6/2
  Freq_MC2/1 -> Divide1/1
  Data Store Read9/1 -> Divide1/3
  Product3/1 -> Add6/1, Subsystem3/1(COMPLD1)
  Data Store Read/1 -> Product3/1
  Add6/1 -> Subsystem3/2(COMPLD2)
  Divide3/1 -> Product1/2, Add1/2
  Freq_MC3/1 -> Divide3/1
  Data Store Read5/1 -> Divide3/3
  Product1/1 -> Add1/1, Subsystem2/1(COMPLD1)
  Divide4/1 -> Product2/2, Add2/2
  Freq_MC4/1 -> Divide4/1
  Data Store Read3/1 -> Divide4/3
  Product2/1 -> Add2/1, Subsystem1/1(COMPLD1)
  Divide2/1 -> Product6/2, Add3/2
  Freq_MC5/1 -> Divide2/1
  Data Store Read13/1 -> Divide2/3
  Product6/1 -> Add3/1, Subsystem/1(COMPLD1)
  Data Store Read1/1 -> Product2/1
  Data Store Read4/1 -> Product1/1
  Data Store Read12/1 -> Product6/1
  Add1/1 -> Subsystem2/2(COMPLD2)
  Add2/1 -> Subsystem1/2(COMPLD2)
  Add3/1 -> Subsystem/2(COMPLD2)
  Pre/1 -> Divide/2
  Pre1/1 -> Divide6/2
  Pre2/1 -> Divide1/2
  Pre3/1 -> Divide2/2
  Pre4/1 -> Divide4/2
  Pre5/1 -> Divide3/2

== system VehCtrl20260630_18B/SigOut/GPIO /HS ==
  note: 3A/5A
  note: 1A/3A
  note: 0.5A/1A
  Data Store Read : DataStoreRead  DataStoreName=HS001
  Data Store Read2 : DataStoreRead  DataStoreName=HS007
  Data Store Read4 : DataStoreRead  DataStoreName=HS002
  Data Store Read5 : DataStoreRead  DataStoreName=HS003
  Data Store Read6 : DataStoreRead  DataStoreName=HS004
  Data Store Read7 : DataStoreRead  DataStoreName=HS005
  Data Store Read9 : DataStoreRead  DataStoreName=HS010
  HS001 : mbd_mpc574x_ec_toolbox/GPIO Blocks/Digital_Output  Priority=1  gpio_pin=PTF5: [SIUL2_GPIO85 | General Purpose IO PF[5]]  gpio_drive_strength=Disabled
  "HS002 " : mbd_mpc574x_ec_toolbox/GPIO Blocks/Digital_Output  Priority=1  gpio_pin=PTF4: [SIUL2_GPIO84 | General Purpose IO PF[4]]  gpio_drive_strength=Disabled
  HS003 : mbd_mpc574x_ec_toolbox/GPIO Blocks/Digital_Output  Priority=1  gpio_pin=PTF3: [SIUL2_GPIO83 | General Purpose IO PF[3]]  gpio_drive_strength=Disabled
  HS004 : mbd_mpc574x_ec_toolbox/GPIO Blocks/Digital_Output  Priority=1  gpio_pin=PTB6: [SIUL2_GPIO22 | General Purpose IO PB[6]]  gpio_drive_strength=Disabled
  HS005 : mbd_mpc574x_ec_toolbox/GPIO Blocks/Digital_Output  Priority=1  gpio_pin=PTA12: [SIUL2_GPIO12 | General Purpose IO PA[12]]  gpio_drive_strength=Disabled
  HS007 : mbd_mpc574x_ec_toolbox/GPIO Blocks/Digital_Output  Priority=1  gpio_pin=PTF7: [SIUL2_GPIO87 | General Purpose IO PF[7]]  gpio_drive_strength=Disabled
  HS010 : mbd_mpc574x_ec_toolbox/GPIO Blocks/Digital_Output  Priority=1  gpio_pin=PTF9: [SIUL2_GPIO89 | General Purpose IO PF[9]]  gpio_drive_strength=Disabled
  wires:
  Data Store Read/1 -> HS001/1
  Data Store Read5/1 -> HS003/1
  Data Store Read4/1 -> "HS002 "/1
  Data Store Read6/1 -> HS004/1
  Data Store Read7/1 -> HS005/1
  Data Store Read2/1 -> HS007/1
  Data Store Read9/1 -> HS010/1

== system VehCtrl20260630_18B/SigOut/GPIO /PWM_OUT ==
  note: LS PWM
  note: HS PWM
  note: Example
  Data Store Read10 : DataStoreRead  DataStoreName=HSO14_PWM_DC
  Data Store Read11 : DataStoreRead  DataStoreName=HSO14_PWM_FRQ
  Data Store Read14 : DataStoreRead  DataStoreName=LSO19_PWM_DC
  Data Store Read15 : DataStoreRead  DataStoreName=LSO19_PWM_FRQ
  Data Store Read2 : DataStoreRead  DataStoreName=HSO08_PWM_DC
  Data Store Read9 : DataStoreRead  DataStoreName=HSO08_PWM_FRQ
  FreqCMD : Stateflow chart  Priority=0  Commented=on  TreatAsAtomicUnit=on
  PWM Configuration and Frequency Update : Subsystem  Commented=on
  PWM Configuration and Frequency Update1 : Subsystem
  PWM Configuration and Frequency Update4 : Subsystem
  wires:
  FreqCMD/1(freq) -> PWM Configuration and Frequency Update/1(In1)
  FreqCMD/2(dc) -> PWM Configuration and Frequency Update/2(In2)
  Data Store Read9/1 -> PWM Configuration and Frequency Update1/2(Fre A)
  Data Store Read2/1 -> PWM Configuration and Frequency Update1/1(PWM A)
  Data Store Read14/1 -> PWM Configuration and Frequency Update4/1(PWM A)
  Data Store Read10/1 -> PWM Configuration and Frequency Update1/3(PWM B)
  Data Store Read11/1 -> PWM Configuration and Frequency Update1/4(Fre B)
  Data Store Read15/1 -> PWM Configuration and Frequency Update4/2(Fre)

== system VehCtrl20260630_18B/SigOut/GPIO /SPI0: LS09_14_15_16_1_2_11_4 ==
  note: 不要开，会重置SPI的初始化设置
  Compare To Constant : simulink/Logic and Bit Operations/Compare To Constant  relop===  const=2  OutDataTypeStr=boolean
  Constant : Constant  OutDataTypeStr=boolean
  Constant1 : Constant  OutDataTypeStr=boolean
  Constant2 : Constant  OutDataTypeStr=boolean
  Data Store Read : DataStoreRead  DataStoreName=VCU_Mode
  Data Store Read1 : DataStoreRead  DataStoreName=SPI0_CS
  LS_CTRL : Subsystem
  LS_CTRL1 : Subsystem
  LS_EN : mbd_mpc574x_ec_toolbox/GPIO Blocks/Digital_Output  Priority=1  gpio_pin=PTA2: [SIUL2_GPIO2 | General Purpose IO PA[2]]  gpio_drive_strength=Disabled
  LS_rst1 : mbd_mpc574x_ec_toolbox/GPIO Blocks/Digital_Output  Priority=1  gpio_pin=PTC10: [SIUL2_GPIO42 | General Purpose IO PC[10]]  gpio_drive_strength=Disabled
  LS_rst2 : mbd_mpc574x_ec_toolbox/GPIO Blocks/Digital_Output  Priority=1  gpio_pin=PTA1: [SIUL2_GPIO1 | General Purpose IO PA[1]]  gpio_drive_strength=Disabled
  Logical Operator : Logic  AllPortsSameDT=off  OutDataTypeStr=boolean
  Logical Operator1 : Logic  Operator=NOT  AllPortsSameDT=off  OutDataTypeStr=boolean
  wires:
  Constant1/1 -> LS_rst2/1
  Constant/1 -> LS_EN/1
  Constant2/1 -> LS_rst1/1
  Data Store Read/1 -> Compare To Constant/1
  Compare To Constant/1 -> Logical Operator/1
  Data Store Read1/1 -> Logical Operator/2
  Logical Operator/1 -> LS_CTRL1/Enable, Logical Operator1/1
  Logical Operator1/1 -> LS_CTRL/Enable

== system VehCtrl20260630_18B/SigOut/GPIO /SPI3: LS03_06_07_08_10_12_13_17_18_19 ==
  Compare To Constant : simulink/Logic and Bit Operations/Compare To Constant  relop===  const=2  OutDataTypeStr=boolean
  Constant1 : Constant  OutDataTypeStr=boolean
  Constant3 : Constant  OutDataTypeStr=boolean
  Data Store Read : DataStoreRead  DataStoreName=VCU_Mode
  Data Store Read3 : DataStoreRead  DataStoreName=SPI3_CS
  LS_EN1 : mbd_mpc574x_ec_toolbox/GPIO Blocks/Digital_Output  Priority=1  gpio_pin=PTF10: [SIUL2_GPIO90 | General Purpose IO PF[10]]  gpio_drive_strength=Disabled
  LS_rst : mbd_mpc574x_ec_toolbox/GPIO Blocks/Digital_Output  Priority=1  gpio_pin=PTC14: [SIUL2_GPIO46 | General Purpose IO PC[14]]  gpio_drive_strength=Disabled
  Logical Operator : Logic  AllPortsSameDT=off  OutDataTypeStr=boolean
  Subsystem : Subsystem
  wires:
  Constant1/1 -> LS_EN1/1
  Constant3/1 -> LS_rst/1
  Data Store Read/1 -> Compare To Constant/1
  Data Store Read3/1 -> Logical Operator/2
  Compare To Constant/1 -> Logical Operator/1
  Logical Operator/1 -> Subsystem/Enable

== system VehCtrl20260630_18B/SigOut/MCU/FL ==
  note: +32
  note: 0-torque
      | 1-speed
  DirCmd : Inport
  torque : Inport  Port=2
  Constant : Constant  Value=16  OutDataTypeStr=uint8
  Constant1 : Constant  Value=4  OutDataTypeStr=uint8
  Constant2 : Constant  Value=DRV_ZEROTURN  OutDataTypeStr=uint8
  Constant3 : Constant  Value=48  OutDataTypeStr=uint8
  Constant4 : Constant  Value=36  OutDataTypeStr=uint8
  Constant5 : Constant  Value=0  OutDataTypeStr=single
  Data Store Read : DataStoreRead  DataStoreName=DrvPhase
  Data Store Read1 : DataStoreRead  DataStoreName=MotorModeZeroTurn
  Data Store Read2 : DataStoreRead  DataStoreName=Gain_Trq2Spd
  GreaterThan : RelationalOperator  Operator===  OutDataTypeStr=boolean  RndMeth=Simplest
  Logical Operator : Logic  AllPortsSameDT=off  OutDataTypeStr=boolean
  NOT : Logic  Operator=NOT  IconShape=distinctive  AllPortsSameDT=off  OutDataTypeStr=boolean
  Product : Product
  Switch{,1..3} (4 alike) : Switch  Criteria=u2 > Threshold
  ModeReq : Outport
  speed : Outport  Port=2
  wires:
  DirCmd/1 -> NOT/1
  Constant/1 -> Switch/1
  Constant1/1 -> Switch/3
  Data Store Read/1 -> GreaterThan/1
  Constant2/1 -> GreaterThan/2
  GreaterThan/1 -> Logical Operator/1
  Data Store Read1/1 -> Logical Operator/2
  Logical Operator/1 -> Switch3/2, Switch1/2
  Switch/1 -> Switch1/3
  Switch1/1 -> ModeReq/1
  NOT/1 -> Switch2/2, Switch/2
  Constant4/1 -> Switch2/3
  Constant3/1 -> Switch2/1
  Switch2/1 -> Switch1/1
  torque/1 -> Product/2
  Switch3/1 -> speed/1
  Product/1 -> Switch3/1
  Data Store Read2/1 -> Product/1
  Constant5/1 -> Switch3/3

== system VehCtrl20260630_18B/SigOut/MCU/FL1 ==
  note: 0-torque
      | 1-speed
  note: +32
  DirCmd : Inport
  torque : Inport  Port=2
  Constant : Constant  Value=16  OutDataTypeStr=uint8
  Constant1 : Constant  Value=4  OutDataTypeStr=uint8
  Constant2 : Constant  Value=DRV_ZEROTURN  OutDataTypeStr=uint8
  Constant3 : Constant  Value=48  OutDataTypeStr=uint8
  Constant4 : Constant  Value=36  OutDataTypeStr=uint8
  Constant5 : Constant  Value=0  OutDataTypeStr=single
  Data Store Read : DataStoreRead  DataStoreName=DrvPhase
  Data Store Read1 : DataStoreRead  DataStoreName=MotorModeZeroTurn
  Data Store Read2 : DataStoreRead  DataStoreName=Gain_Trq2Spd
  GreaterThan : RelationalOperator  Operator===  OutDataTypeStr=boolean  RndMeth=Simplest
  Logical Operator : Logic  AllPortsSameDT=off  OutDataTypeStr=boolean
  NOT : Logic  Operator=NOT  IconShape=distinctive  AllPortsSameDT=off  OutDataTypeStr=boolean
  Product : Product
  Switch{,1..3} (4 alike) : Switch  Criteria=u2 > Threshold
  ModeReq : Outport
  speed : Outport  Port=2
  wires:
  Constant5/1 -> Switch3/3
  Data Store Read2/1 -> Product/1
  Product/1 -> Switch3/1
  Switch3/1 -> speed/1
  torque/1 -> Product/2
  Switch2/1 -> Switch1/1
  Constant3/1 -> Switch2/1
  Constant4/1 -> Switch2/3
  NOT/1 -> Switch/2, Switch2/2
  Switch1/1 -> ModeReq/1
  Switch/1 -> Switch1/3
  Logical Operator/1 -> Switch1/2, Switch3/2
  Data Store Read1/1 -> Logical Operator/2
  GreaterThan/1 -> Logical Operator/1
  Constant2/1 -> GreaterThan/2
  Data Store Read/1 -> GreaterThan/1
  Constant1/1 -> Switch/3
  Constant/1 -> Switch/1
  DirCmd/1 -> NOT/1

== system VehCtrl20260630_18B/SigOut/MCU/FL2 ==
  note: +32
  note: 0-torque
      | 1-speed
  DirCmd : Inport
  torque : Inport  Port=2
  Constant : Constant  Value=16  OutDataTypeStr=uint8
  Constant1 : Constant  Value=4  OutDataTypeStr=uint8
  Constant2 : Constant  Value=DRV_ZEROTURN  OutDataTypeStr=uint8
  Constant3 : Constant  Value=48  OutDataTypeStr=uint8
  Constant4 : Constant  Value=36  OutDataTypeStr=uint8
  Constant5 : Constant  Value=0  OutDataTypeStr=single
  Data Store Read : DataStoreRead  DataStoreName=DrvPhase
  Data Store Read1 : DataStoreRead  DataStoreName=MotorModeZeroTurn
  Data Store Read2 : DataStoreRead  DataStoreName=Gain_Trq2Spd
  GreaterThan : RelationalOperator  Operator===  OutDataTypeStr=boolean  RndMeth=Simplest
  Logical Operator : Logic  AllPortsSameDT=off  OutDataTypeStr=boolean
  Product : Product
  Switch{,1..3} (4 alike) : Switch  Criteria=u2 > Threshold
  ModeReq : Outport
  speed : Outport  Port=2
  wires:
  Constant/1 -> Switch/1
  Constant1/1 -> Switch/3
  Data Store Read/1 -> GreaterThan/1
  Constant2/1 -> GreaterThan/2
  GreaterThan/1 -> Logical Operator/1
  Data Store Read1/1 -> Logical Operator/2
  Logical Operator/1 -> Switch3/2, Switch1/2
  Switch/1 -> Switch1/3
  Switch1/1 -> ModeReq/1
  DirCmd/1 -> Switch2/2, Switch/2
  Constant4/1 -> Switch2/3
  Constant3/1 -> Switch2/1
  Switch2/1 -> Switch1/1
  torque/1 -> Product/2
  Switch3/1 -> speed/1
  Product/1 -> Switch3/1
  Data Store Read2/1 -> Product/1
  Constant5/1 -> Switch3/3
